simulink model "nnadaptive"  (R2024a)
settings: Solver=VariableStepAuto  StartTime=0.0  StopTime=10  RelTol=1e-3
settings Model: Creator=ericliu  LastModifiedBy=Eason

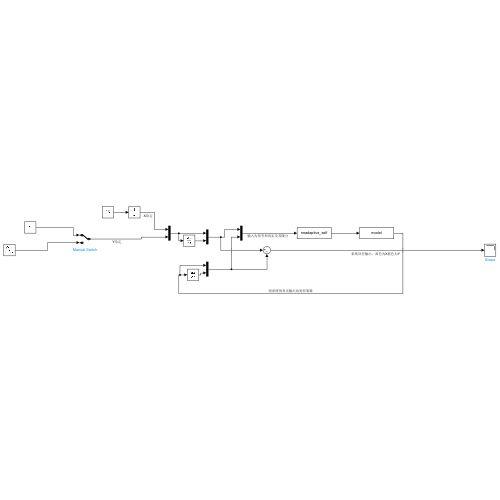
[thumbnail: Simulink's stored preview of the top-level diagram]
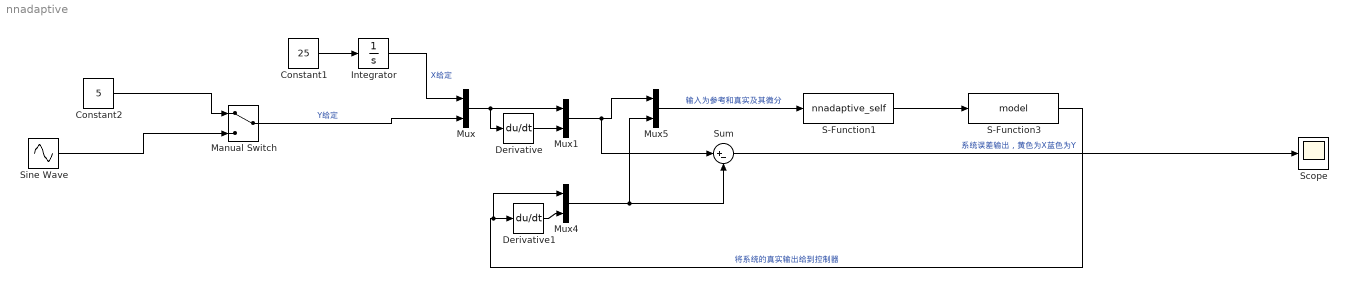
== system nnadaptive ==
  Constant1 : Constant  Value=25  SampleTime=0.001
  Constant2 : Constant  Value=5
  Derivative : Derivative
  Derivative1 : Derivative
  Integrator : Integrator
  Manual Switch : ManualSwitch
  Mux{,1,4..5} (4 alike) : Mux  Inputs=2
  S-Function1 : S-Function  FunctionName=nnadaptive_self  SFunctionDeploymentMode=off  EnableBusSupport=off
  S-Function3 : S-Function  FunctionName=model  SFunctionDeploymentMode=off  EnableBusSupport=off
  Scope : Scope
  Sine Wave : Sin  Amplitude=4  Frequency=0.5  SampleTime=0
  Sum : Sum  Inputs=|+-
  wires:
  Mux/1 -> Derivative/1, Mux1/1
  Derivative/1 -> Mux1/2
  Derivative1/1 -> Mux4/2
  S-Function3/1 -> Derivative1/1, Mux4/1  "将系统的真实输出给到控制器"
  Mux4/1 -> Sum/2, Mux5/2
  S-Function1/1 -> S-Function3/1
  Mux5/1 -> S-Function1/1  "输入为参考和真实及其微分"
  Mux1/1 -> Sum/1, Mux5/1
  Sum/1 -> Scope/1  "系统误差输出，黄色为X蓝色为Y"
  Constant1/1 -> Integrator/1
  Integrator/1 -> Mux/1  "X给定"
  Constant2/1 -> Manual Switch/1
  Manual Switch/1 -> Mux/2  "Y给定"
  Sine Wave/1 -> Manual Switch/2
